simulink model "Record_accelerometer"  (R2014a)
settings: Solver=FixedStepDiscrete  StartTime=0.0  StopTime=300  FixedStep=1/400  RelTol=1e-3
undefined symbols (not defined in the file or in its folder): DiscIntNeverNeededParam
libraries: simulink x6, aerolibtransform2 x4, vrlib x3, aerolibutil x2, AR_Drone_2_Library x1, dspmtrx3 x1, Navigation_Lib x1
(part 2 of 2)

== system Record_accelerometer/Navigation Subsystem/CheckSum Pre-Processing/RateGyro Processing/CheckSum Correction ==
  CalculatedData : Inport
  CheckSumFlag : Inport  Port=2
  Holding Value : Inport  Port=3
  Compare To Zero : simulink/Logic and Bit Operations/Compare To Zero  relop=>  OutDataTypeStr=boolean
  Delay : Delay  DelayLength=3  InitialCondition=0
  Generate Sample Holding Pulse : Subsystem
  "If True, we have good data, If false, we have bad data, With bad data, use previous good data from N samples ago and hold it on that value for M samples" : Switch  Criteria=u2 > Threshold
  Invert Logic : Logic  Operator=NOT  AllPortsSameDT=off  OutDataTypeStr=boolean
  Logical Operator1 : Logic  Operator=NOT  AllPortsSameDT=off  OutDataTypeStr=boolean
  Pre-Processed Height : Outport
  wires:
  CheckSumFlag/1 -> Compare To Zero/1
  CalculatedData/1 -> "If True, we have good data, If false, we have bad data, With bad data, use previous good data from N samples ago and hold it on that value for M samples"/1
  "If True, we have good data, If false, we have bad data, With bad data, use previous good data from N samples ago and hold it on that value for M samples"/1 -> Pre-Processed Height/1, Delay/1
  Delay/1 -> "If True, we have good data, If false, we have bad data, With bad data, use previous good data from N samples ago and hold it on that value for M samples"/3
  Compare To Zero/1 -> Logical Operator1/1
  Generate Sample Holding Pulse/1(Hold_Data_Pulse) -> Invert Logic/1
  Logical Operator1/1 -> Generate Sample Holding Pulse/1(CheckSumFlag)
  Invert Logic/1 -> "If True, we have good data, If false, we have bad data, With bad data, use previous good data from N samples ago and hold it on that value for M samples"/2
  Holding Value/1 -> Generate Sample Holding Pulse/2(HoldDataTicks_Value)

== system Record_accelerometer/Navigation Subsystem/CheckSum Pre-Processing/RateGyro Processing/Process Data ==
  note: const float Sensitivity[ 3 ] = { 0.0609 , 0.0609 , 0.0609 } ;
      | const float Neutral[ 3 ] = { 0.0 , 0.0 , 0.0 } ;
      | const int16_t Offset[ 3 ] = { - 73 , 14 , - 13 } ;
      | const int16_t Noises[ 3 ] = { 35 , 35 , 15 } ;
      |
      | int16_t vRaws[ 3 ] = {
      | Navdata :: IMU :: Gyroscope :: getRawX (),
      | Navdata :: IMU :: Gyroscope :: getRawY (),
      | Navdata :: IMU :: Gyroscope :: getRawZ ()
      | } ;
      |
      | gyroscope[i] = vRaws[i] * Gyroscope :: Sensitivity[i] * M_PI / 180.0 ;
  Raw Data : Inport
  Constant : Constant  Value=[0.0, 0.0, 0.0]
  Gain : Gain  Gain=[0.0609, 0.0609, 0.0609]
  Sum : Sum  Inputs=|++
  Processed Data : Outport
  wires:
  Sum/1 -> Gain/1
  Gain/1 -> Processed Data/1
  Constant/1 -> Sum/2
  Raw Data/1 -> Sum/1

== system Record_accelerometer/Navigation Subsystem/CheckSum Pre-Processing/TempFilter/CheckSum Correction ==
  CalculatedData : Inport
  CheckSumFlag : Inport  Port=2
  Holding Value : Inport  Port=3
  Compare To Zero : simulink/Logic and Bit Operations/Compare To Zero  relop=>  OutDataTypeStr=boolean
  Delay : Delay  DelayLength=3  InitialCondition=0
  Generate Sample Holding Pulse : Subsystem
  "If True, we have good data, If false, we have bad data, With bad data, use previous good data from N samples ago and hold it on that value for M samples" : Switch  Criteria=u2 > Threshold
  Invert Logic : Logic  Operator=NOT  AllPortsSameDT=off  OutDataTypeStr=boolean
  Logical Operator1 : Logic  Operator=NOT  AllPortsSameDT=off  OutDataTypeStr=boolean
  Pre-Processed Data : Outport
  wires:
  CheckSumFlag/1 -> Compare To Zero/1
  CalculatedData/1 -> "If True, we have good data, If false, we have bad data, With bad data, use previous good data from N samples ago and hold it on that value for M samples"/1
  "If True, we have good data, If false, we have bad data, With bad data, use previous good data from N samples ago and hold it on that value for M samples"/1 -> Pre-Processed Data/1, Delay/1
  Delay/1 -> "If True, we have good data, If false, we have bad data, With bad data, use previous good data from N samples ago and hold it on that value for M samples"/3
  Compare To Zero/1 -> Logical Operator1/1
  Generate Sample Holding Pulse/1(Hold_Data_Pulse) -> Invert Logic/1
  Logical Operator1/1 -> Generate Sample Holding Pulse/1(CheckSumFlag)
  Invert Logic/1 -> "If True, we have good data, If false, we have bad data, With bad data, use previous good data from N samples ago and hold it on that value for M samples"/2
  Holding Value/1 -> Generate Sample Holding Pulse/2(HoldDataTicks_Value)

== system Record_accelerometer/Navigation Subsystem/CheckSum Pre-Processing/TempFilter/Process Raw Mag Data ==
  note: magnetometer[ 0 ] = - ( float ) navdata.mx ;
      | magnetometer[ 1 ] = ( float ) navdata.my ;
      | magnetometer[ 2 ] = - ( float ) navdata.mz ;
      | const float Sensitivity[ 3 ] = { 0.0071492608 , 0.0070882491 , 0.0074057781 } ;
      | const float Neutral[ 3 ] = { 118.0 , - 65.0 , 110.0 } ;
  Magnetometer : Inport
  Bias : Constant  Value=[ 118.0, -65.0, 110.0 ]
  Sum : Sum  Inputs=|+-
  postGain : Gain  Gain=[0.0071492608, 0.0070882491, 0.0074057781]
  preGain : Gain  Gain=[-1 1 -1]
  ProcessedData : Outport
  wires:
  postGain/1 -> ProcessedData/1
  Magnetometer/1 -> preGain/1
  Sum/1 -> postGain/1
  preGain/1 -> Sum/1
  Bias/1 -> Sum/2

== system Record_accelerometer/Navigation Subsystem/CheckSum Pre-Processing/TempFilter1/CheckSum Correction ==
  CalculatedData : Inport
  CheckSumFlag : Inport  Port=2
  Holding Value : Inport  Port=3
  Compare To Zero : simulink/Logic and Bit Operations/Compare To Zero  relop=>  OutDataTypeStr=boolean
  Delay : Delay  DelayLength=3  InitialCondition=0
  Generate Sample Holding Pulse : Subsystem
  "If True, we have good data, If false, we have bad data, With bad data, use previous good data from N samples ago and hold it on that value for M samples" : Switch  Criteria=u2 > Threshold
  Invert Logic : Logic  Operator=NOT  AllPortsSameDT=off  OutDataTypeStr=boolean
  Logical Operator1 : Logic  Operator=NOT  AllPortsSameDT=off  OutDataTypeStr=boolean
  Pre-Processed Data : Outport
  wires:
  CheckSumFlag/1 -> Compare To Zero/1
  CalculatedData/1 -> "If True, we have good data, If false, we have bad data, With bad data, use previous good data from N samples ago and hold it on that value for M samples"/1
  "If True, we have good data, If false, we have bad data, With bad data, use previous good data from N samples ago and hold it on that value for M samples"/1 -> Pre-Processed Data/1, Delay/1
  Delay/1 -> "If True, we have good data, If false, we have bad data, With bad data, use previous good data from N samples ago and hold it on that value for M samples"/3
  Compare To Zero/1 -> Logical Operator1/1
  Generate Sample Holding Pulse/1(Hold_Data_Pulse) -> Invert Logic/1
  Logical Operator1/1 -> Generate Sample Holding Pulse/1(CheckSumFlag)
  Invert Logic/1 -> "If True, we have good data, If false, we have bad data, With bad data, use previous good data from N samples ago and hold it on that value for M samples"/2
  Holding Value/1 -> Generate Sample Holding Pulse/2(HoldDataTicks_Value)

== system Record_accelerometer/Navigation Subsystem/CheckSum Pre-Processing/TempFilter1/Process Raw Mag Data ==
  note: magnetometer[ 0 ] = - ( float ) navdata.mx ;
      | magnetometer[ 1 ] = ( float ) navdata.my ;
      | magnetometer[ 2 ] = - ( float ) navdata.mz ;
      | const float Sensitivity[ 3 ] = { 0.0071492608 , 0.0070882491 , 0.0074057781 } ;
      | const float Neutral[ 3 ] = { 118.0 , - 65.0 , 110.0 } ;
  Magnetometer : Inport
  Bias : Constant  Value=[ 118.0, -65.0, 110.0 ]
  Sum : Sum  Inputs=|+-
  postGain : Gain  Gain=[0.0071492608, 0.0070882491, 0.0074057781]
  preGain : Gain  Gain=[-1 1 -1]
  ProcessedData : Outport
  wires:
  postGain/1 -> ProcessedData/1
  Magnetometer/1 -> preGain/1
  Sum/1 -> postGain/1
  preGain/1 -> Sum/1
  Bias/1 -> Sum/2

== system Record_accelerometer/Navigation Subsystem/CheckSum Pre-Processing/Ultrasound Processing/CheckSum Correction ==
  CalculatedData : Inport
  CheckSumFlag : Inport  Port=2
  Holding Value : Inport  Port=3
  Compare To Zero : simulink/Logic and Bit Operations/Compare To Zero  relop=>  OutDataTypeStr=boolean
  Delay : Delay  DelayLength=3  InitialCondition=0
  Generate Sample Holding Pulse : Subsystem
  "If True, we have good data, If false, we have bad data, With bad data, use previous good data from N samples ago and hold it on that value for M samples" : Switch  Criteria=u2 > Threshold
  Invert Logic : Logic  Operator=NOT  AllPortsSameDT=off  OutDataTypeStr=boolean
  Logical Operator1 : Logic  Operator=NOT  AllPortsSameDT=off  OutDataTypeStr=boolean
  Pre-Processed Height : Outport
  wires:
  CheckSumFlag/1 -> Compare To Zero/1
  CalculatedData/1 -> "If True, we have good data, If false, we have bad data, With bad data, use previous good data from N samples ago and hold it on that value for M samples"/1
  "If True, we have good data, If false, we have bad data, With bad data, use previous good data from N samples ago and hold it on that value for M samples"/1 -> Pre-Processed Height/1, Delay/1
  Delay/1 -> "If True, we have good data, If false, we have bad data, With bad data, use previous good data from N samples ago and hold it on that value for M samples"/3
  Compare To Zero/1 -> Logical Operator1/1
  Generate Sample Holding Pulse/1(Hold_Data_Pulse) -> Invert Logic/1
  Logical Operator1/1 -> Generate Sample Holding Pulse/1(CheckSumFlag)
  Invert Logic/1 -> "If True, we have good data, If false, we have bad data, With bad data, use previous good data from N samples ago and hold it on that value for M samples"/2
  Holding Value/1 -> Generate Sample Holding Pulse/2(HoldDataTicks_Value)

== system Record_accelerometer/Navigation Subsystem/Remove Temperature Gyro Offset/TemperatureOffset (home_330453)/Convert to Celcius ==
  In1 : Inport
  Constant1 : Constant  Value=23000  OutDataTypeStr=int16
  Data Type Conversion3 : DataTypeConversion  OutDataTypeStr=int16
  Gain1 : Gain  Gain=1/280  OutDataTypeStr=double
  Sum4 : Sum  Inputs=|++
  Out1 : Outport
  wires:
  Sum4/1 -> Gain1/1
  Gain1/1 -> Out1/1
  In1/1 -> Data Type Conversion3/1
  Data Type Conversion3/1 -> Sum4/1
  Constant1/1 -> Sum4/2

== system Record_accelerometer/Navigation Subsystem/Remove Temperature Gyro Offset/TemperatureOffset (home_330453)/Temperature Correct Pitch ==
  Temp : Inport
  Constant : Constant  Value=-293.2
  Data Type Conversion : DataTypeConversion  OutDataTypeStr=int16
  Gain1 : Gain  Commented=through  Gain=0.01074
  Gain2 : Gain  Gain=0.005239
  Sum : Sum  Inputs=|++
  Offset Correct : Outport
  wires:
  Gain2/1 -> Gain1/1
  Constant/1 -> Sum/2
  Sum/1 -> Data Type Conversion/1
  Gain1/1 -> Sum/1
  Temp/1 -> Gain2/1
  Data Type Conversion/1 -> Offset Correct/1

== system Record_accelerometer/Navigation Subsystem/Remove Temperature Gyro Offset/TemperatureOffset (home_330453)/Temperature Correct Pitch1 ==
  note: % Linear model Poly2:
      | %      f(x) = p1*x^2 + p2*x + p3
      | % Coefficients (with 95% confidence bounds):
      | %        p1 =    0.006948  (0.006782, 0.007115)
      | %        p2 =       1.056  (1.041, 1.071)
      | %        p3 =      -66.21  (-66.54, -65.88)
  Temp : Inport
  Constant1 : Constant  Value=4.961
  Gain : Gain  Gain=0.009828
  Gain3 : Gain  Gain=0.4486
  Product : Product
  Sum1 : Sum  Inputs=|+++
  Offset Correct : Outport
  wires:
  Temp/1 -> Product/1, Gain3/1, Product/2
  Product/1 -> Gain/1
  Gain/1 -> Sum1/1
  Gain3/1 -> Sum1/2
  Constant1/1 -> Sum1/3
  Sum1/1 -> Offset Correct/1

== system Record_accelerometer/Navigation Subsystem/Remove Temperature Gyro Offset/TemperatureOffset (home_330453)/Temperature Correct Roll ==
  Temp : Inport
  Data Type Conversion : DataTypeConversion  OutDataTypeStr=int16
  Offset : Constant  Value=-498.8
  Slope : Gain  Gain=0.01074
  Sum : Sum  Inputs=|++
  Offset Correction : Outport
  wires:
  Data Type Conversion/1 -> Offset Correction/1
  Offset/1 -> Sum/2
  Sum/1 -> Data Type Conversion/1  "Temperature Offset Correction"
  Slope/1 -> Sum/1
  Temp/1 -> Slope/1

== system Record_accelerometer/Navigation Subsystem/Remove Temperature Gyro Offset/TemperatureOffset (home_330453)/Temperature Correct Roll1 ==
  note: f(x) = p1*x^2 + p2*x + p3
      | Coefficients (with 95% confidence bounds):
      |        p1 =     0.01851  (0.0183, 0.01872)
      |        p2 =       1.553  (1.534, 1.572)
      |        p3 =      -13.59  (-14, -13.17)
  Temp : Inport
  Constant : Constant  Commented=on  Value=-47.33
  Constant1 : Constant  Value=-72.51+5
  Gain : Gain  Gain=-0.004462
  Gain1 : Gain  Commented=through  Gain=0.01074
  Gain2 : Gain  Commented=through  Gain=3.139
  Gain3 : Gain  Gain=1.144
  Product : Product
  Sum : Sum  Inputs=|++
  Sum1 : Sum  Inputs=|+++
  Offset Correct : Outport
  wires:
  Gain2/1 -> Gain1/1
  Constant/1 -> Sum/2
  Sum/1 -> Product/1, Gain3/1, Product/2
  Gain1/1 -> Sum/1
  Temp/1 -> Gain2/1
  Product/1 -> Gain/1
  Gain/1 -> Sum1/1
  Gain3/1 -> Sum1/2
  Constant1/1 -> Sum1/3
  Sum1/1 -> Offset Correct/1

== system Record_accelerometer/Navigation Subsystem/Remove Temperature Gyro Offset/TemperatureOffset (home_330453)/Temperature Correct Yaw ==
  Temp : Inport
  Constant : Constant  Value=-40.65
  Data Type Conversion : DataTypeConversion  OutDataTypeStr=int16
  Gain1 : Gain  Commented=through  Gain=0.01074
  Gain2 : Gain  Gain=0.0008992
  Sum : Sum  Inputs=|++
  Offset Correct : Outport
  wires:
  Gain2/1 -> Gain1/1
  Constant/1 -> Sum/2
  Sum/1 -> Data Type Conversion/1
  Gain1/1 -> Sum/1
  Temp/1 -> Gain2/1
  Data Type Conversion/1 -> Offset Correct/1

== system Record_accelerometer/Navigation Subsystem/Remove Temperature Gyro Offset/TemperatureOffset (home_330453)/Temperature Correct Yaw1 ==
  note: f(x) = p1*x^2 + p2*x + p3
      | Coefficients (with 95% confidence bounds):
      |        p1 =     0.01851  (0.0183, 0.01872)
      |        p2 =       1.553  (1.534, 1.572)
      |        p3 =      -13.59  (-14, -13.17)
  note: f(x) = p1*x^2 + p2*x + p3
      | Coefficients (with 95% confidence bounds):
      |        p1 =    -0.00233  (-0.002509, -0.00215)
      |        p2 =        0.46  (0.444, 0.476)
      |        p3 =      -7.059  (-7.413, -6.705)
  Temp : Inport
  Constant : Constant  Commented=on  Value=-47.33
  Constant1 : Constant  Value=-7.059
  Gain : Gain  Gain=-0.00233
  Gain1 : Gain  Commented=through  Gain=0.01074
  Gain2 : Gain  Commented=through  Gain=3.139
  Gain3 : Gain  Gain=0.46
  Product : Product
  Sum : Sum  Inputs=|++
  Sum1 : Sum  Inputs=|+++
  Offset Correct : Outport
  wires:
  Gain2/1 -> Gain1/1
  Constant/1 -> Sum/2
  Sum/1 -> Product/1, Gain3/1, Product/2
  Gain1/1 -> Sum/1
  Temp/1 -> Gain2/1
  Product/1 -> Gain/1
  Gain/1 -> Sum1/1
  Gain3/1 -> Sum1/2
  Constant1/1 -> Sum1/3
  Sum1/1 -> Offset Correct/1

== system Record_accelerometer/Navigation Subsystem/Remove Temperature Gyro Offset/TemperatureOffset (work_255725)/Convert to Celcius ==
  In1 : Inport
  Constant1 : Constant  Value=23000  OutDataTypeStr=int16
  Data Type Conversion3 : DataTypeConversion  OutDataTypeStr=int16
  Gain1 : Gain  Gain=1/280  OutDataTypeStr=double
  Sum4 : Sum  Inputs=|++
  Out1 : Outport
  wires:
  Sum4/1 -> Gain1/1
  Gain1/1 -> Out1/1
  In1/1 -> Data Type Conversion3/1
  Data Type Conversion3/1 -> Sum4/1
  Constant1/1 -> Sum4/2

== system Record_accelerometer/Navigation Subsystem/Remove Temperature Gyro Offset/TemperatureOffset (work_255725)/Temperature Correct Pitch ==
  Temp : Inport
  Constant : Constant  Value=-293.2
  Data Type Conversion : DataTypeConversion  OutDataTypeStr=int16
  Gain1 : Gain  Commented=through  Gain=0.01074
  Gain2 : Gain  Gain=0.005239
  Sum : Sum  Inputs=|++
  Offset Correct : Outport
  wires:
  Gain2/1 -> Gain1/1
  Constant/1 -> Sum/2
  Sum/1 -> Data Type Conversion/1
  Gain1/1 -> Sum/1
  Temp/1 -> Gain2/1
  Data Type Conversion/1 -> Offset Correct/1

== system Record_accelerometer/Navigation Subsystem/Remove Temperature Gyro Offset/TemperatureOffset (work_255725)/Temperature Correct Pitch1 ==
  note: % Linear model Poly2:
      | %      f(x) = p1*x^2 + p2*x + p3
      | % Coefficients (with 95% confidence bounds):
      | %        p1 =    0.006948  (0.006782, 0.007115)
      | %        p2 =       1.056  (1.041, 1.071)
      | %        p3 =      -66.21  (-66.54, -65.88)
  Temp : Inport
  Constant1 : Constant  Value=-66.21
  Gain : Gain  Gain=0.006948
  Gain3 : Gain  Gain=1.056
  Product : Product
  Sum1 : Sum  Inputs=|+++
  Offset Correct : Outport
  wires:
  Temp/1 -> Product/1, Gain3/1, Product/2
  Product/1 -> Gain/1
  Gain/1 -> Sum1/1
  Gain3/1 -> Sum1/2
  Constant1/1 -> Sum1/3
  Sum1/1 -> Offset Correct/1

== system Record_accelerometer/Navigation Subsystem/Remove Temperature Gyro Offset/TemperatureOffset (work_255725)/Temperature Correct Roll ==
  Temp : Inport
  Data Type Conversion : DataTypeConversion  OutDataTypeStr=int16
  Offset : Constant  Value=-498.8
  Slope : Gain  Gain=0.01074
  Sum : Sum  Inputs=|++
  Offset Correction : Outport
  wires:
  Data Type Conversion/1 -> Offset Correction/1
  Offset/1 -> Sum/2
  Sum/1 -> Data Type Conversion/1  "Temperature Offset Correction"
  Slope/1 -> Sum/1
  Temp/1 -> Slope/1

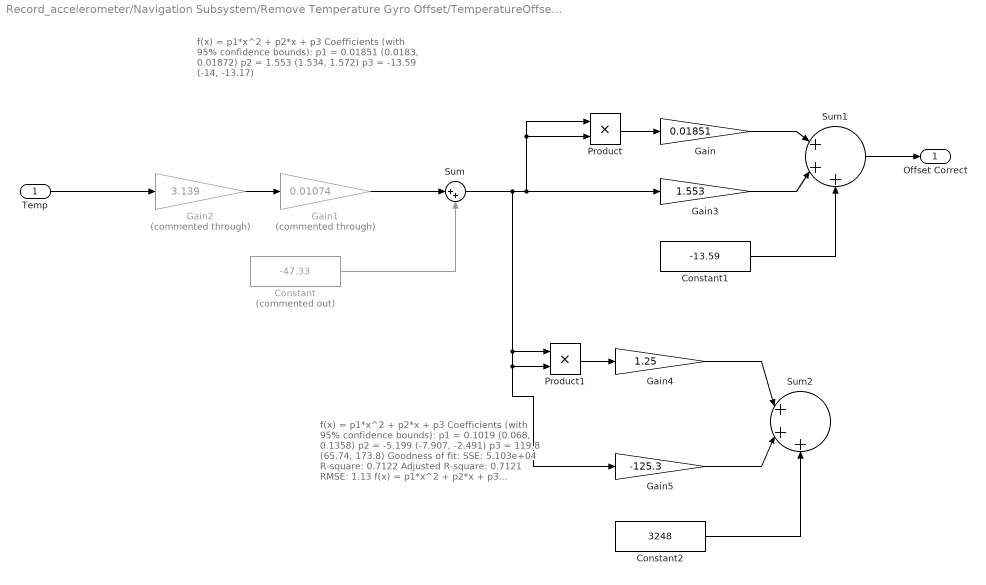
== system Record_accelerometer/Navigation Subsystem/Remove Temperature Gyro Offset/TemperatureOffset (work_255725)/Temperature Correct Roll1 ==
  note: f(x) = p1*x^2 + p2*x + p3
      | Coefficients (with 95% confidence bounds):
      |        p1 =      0.1019  (0.068, 0.1358)
      |        p2 =      -5.199  (-7.907, -2.491)
      |        p3 =       119.8  (65.74, 173.8)
      |
      | Goodness of fit:
      |   SSE: 5.103e+04
      |   R-square: 0.7122
      |   Adjusted R-square: 0.7121
      |   RMSE: 1.13
      |
      |
      |      f(x) = p1*x^2 + p2*x + p3
      | Coefficients (with 95% confidence bounds):
      |        p1 =        1.25  (1.214, 1.287)
      |        p2 =      -125.3  (-129.1, -121.5)
      |        p3 =        3248  (3149, 3347)
  note: f(x) = p1*x^2 + p2*x + p3
      | Coefficients (with 95% confidence bounds):
      |        p1 =     0.01851  (0.0183, 0.01872)
      |        p2 =       1.553  (1.534, 1.572)
      |        p3 =      -13.59  (-14, -13.17)
  Temp : Inport
  Constant : Constant  Commented=on  Value=-47.33
  Constant1 : Constant  Value=-13.59
  Constant2 : Constant  Value=3248
  Gain : Gain  Gain=0.01851
  Gain1 : Gain  Commented=through  Gain=0.01074
  Gain2 : Gain  Commented=through  Gain=3.139
  Gain3 : Gain  Gain=1.553
  Gain4 : Gain  Gain=1.25
  Gain5 : Gain  Gain=-125.3
  Product : Product
  Product1 : Product
  Sum : Sum  Inputs=|++
  Sum1 : Sum  Inputs=|+++
  Sum2 : Sum  Inputs=|+++
  Offset Correct : Outport
  wires:
  Gain2/1 -> Gain1/1
  Constant/1 -> Sum/2
  Sum/1 -> Product/2, Product/1, Gain3/1, Product1/1, Gain5/1, Product1/2
  Gain1/1 -> Sum/1
  Temp/1 -> Gain2/1
  Product/1 -> Gain/1
  Gain/1 -> Sum1/1
  Gain3/1 -> Sum1/2
  Constant1/1 -> Sum1/3
  Gain4/1 -> Sum2/1
  Gain5/1 -> Sum2/2
  Constant2/1 -> Sum2/3
  Product1/1 -> Gain4/1
  Sum1/1 -> Offset Correct/1

== system Record_accelerometer/Navigation Subsystem/Remove Temperature Gyro Offset/TemperatureOffset (work_255725)/Temperature Correct Yaw ==
  Temp : Inport
  Constant : Constant  Value=-40.65
  Data Type Conversion : DataTypeConversion  OutDataTypeStr=int16
  Gain1 : Gain  Commented=through  Gain=0.01074
  Gain2 : Gain  Gain=0.0008992
  Sum : Sum  Inputs=|++
  Offset Correct : Outport
  wires:
  Gain2/1 -> Gain1/1
  Constant/1 -> Sum/2
  Sum/1 -> Data Type Conversion/1
  Gain1/1 -> Sum/1
  Temp/1 -> Gain2/1
  Data Type Conversion/1 -> Offset Correct/1

== system Record_accelerometer/Navigation Subsystem/Remove Temperature Gyro Offset/TemperatureOffset (work_255725)/Temperature Correct Yaw1 ==
  note: f(x) = p1*x^2 + p2*x + p3
      | Coefficients (with 95% confidence bounds):
      |        p1 =     0.01851  (0.0183, 0.01872)
      |        p2 =       1.553  (1.534, 1.572)
      |        p3 =      -13.59  (-14, -13.17)
  note: f(x) = p1*x^2 + p2*x + p3
      | Coefficients (with 95% confidence bounds):
      |        p1 =    -0.00233  (-0.002509, -0.00215)
      |        p2 =        0.46  (0.444, 0.476)
      |        p3 =      -7.059  (-7.413, -6.705)
  Temp : Inport
  Constant : Constant  Commented=on  Value=-47.33
  Constant1 : Constant  Value=-7.962
  Gain : Gain  Gain=0.009834
  Gain1 : Gain  Commented=through  Gain=0.01074
  Gain2 : Gain  Commented=through  Gain=3.139
  Gain3 : Gain  Gain=-0.4009
  Product : Product
  Sum : Sum  Inputs=|++
  Sum1 : Sum  Inputs=|+++
  Offset Correct : Outport
  wires:
  Gain2/1 -> Gain1/1
  Constant/1 -> Sum/2
  Sum/1 -> Product/1, Gain3/1, Product/2
  Gain1/1 -> Sum/1
  Temp/1 -> Gain2/1
  Product/1 -> Gain/1
  Gain/1 -> Sum1/1
  Gain3/1 -> Sum1/2
  Constant1/1 -> Sum1/3
  Sum1/1 -> Offset Correct/1

== system Record_accelerometer/Navigation Subsystem/Remove Temperature Gyro Offset/TemperatureOffset (work_255725)/Temperature Correct Yaw2 ==
  note: f(x) = p1*x^2 + p2*x + p3
      | Coefficients (with 95% confidence bounds):
      |        p1 =     0.01851  (0.0183, 0.01872)
      |        p2 =       1.553  (1.534, 1.572)
      |        p3 =      -13.59  (-14, -13.17)
  note: f(x) = p1*x^2 + p2*x + p3
      | Coefficients (with 95% confidence bounds):
      |        p1 =    -0.00233  (-0.002509, -0.00215)
      |        p2 =        0.46  (0.444, 0.476)
      |        p3 =      -7.059  (-7.413, -6.705)
  Temp : Inport
  Constant : Constant  Commented=on  Value=-47.33
  Constant1 : Constant  Value=-7.059
  Gain : Gain  Gain=-0.00233
  Gain1 : Gain  Commented=through  Gain=0.01074
  Gain2 : Gain  Commented=through  Gain=3.139
  Gain3 : Gain  Gain=0.46
  Product : Product
  Sum : Sum  Inputs=|++
  Sum1 : Sum  Inputs=|+++
  Offset Correct : Outport
  wires:
  Gain2/1 -> Gain1/1
  Constant/1 -> Sum/2
  Sum/1 -> Product/1, Gain3/1, Product/2
  Gain1/1 -> Sum/1
  Temp/1 -> Gain2/1
  Product/1 -> Gain/1
  Gain/1 -> Sum1/1
  Gain3/1 -> Sum1/2
  Constant1/1 -> Sum1/3
  Sum1/1 -> Offset Correct/1

== system Record_accelerometer/Navigation Subsystem/SL3D Visualization/Interchange Axes Mag for SL3D /Home Drone ==
  note: This comes close, however, it doesnt seem that the axis changes properly
      | ie: i rotate drone, the green dot follows it. This  tells me the Z-axis is not
      |  properly placed
  note: y
  note: x
  note: z
  In1 : Inport
  Demux1 : Demux  Outputs=3
  Gain : Gain  Gain=-1
  Gain1 : Gain
  Gain2 : Gain
  Mux2 : Mux  Inputs=3
  Out1 : Outport
  wires:
  Mux2/1 -> Out1/1
  In1/1 -> Demux1/1
  Demux1/3 -> Gain2/1
  Gain2/1 -> Mux2/2
  Demux1/1 -> Gain/1
  Gain/1 -> Mux2/3
  Demux1/2 -> Gain1/1
  Gain1/1 -> Mux2/1

== system Record_accelerometer/Navigation Subsystem/SL3D Visualization/Interchange Axes Mag for SL3D /Subsystem ==
  note: This comes close, however, it doesnt seem that the axis changes properly
      | ie: i rotate drone, the green dot follows it. This  tells me the Z-axis is not
      |  properly placed
  note: y
  note: x
  note: z
  In1 : Inport
  Demux1 : Demux  Outputs=3
  Gain : Gain
  Gain1 : Gain  Gain=-1
  Gain2 : Gain  Gain=-1
  Mux2 : Mux  Inputs=3
  Out1 : Outport
  wires:
  Demux1/1 -> Gain2/1
  Gain2/1 -> Mux2/2
  Gain/1 -> Mux2/3
  Gain1/1 -> Mux2/1
  Mux2/1 -> Out1/1
  Demux1/2 -> Gain1/1
  Demux1/3 -> Gain/1
  In1/1 -> Demux1/1

== system Record_accelerometer/Navigation Subsystem/SL3D Visualization/Interchange Axes Mag for SL3D /Work Drone ==
  note: This comes close, however, it doesnt seem that the axis changes properly
      | ie: i rotate drone, the green dot follows it. This  tells me the Z-axis is not
      |  properly placed
  note: y
  note: x
  note: z
  In1 : Inport
  Demux1 : Demux  Outputs=3
  Gain : Gain  Gain=-1
  Gain1 : Gain
  Gain2 : Gain
  Mux2 : Mux  Inputs=3
  Out1 : Outport
  wires:
  Mux2/1 -> Out1/1
  In1/1 -> Demux1/1
  Demux1/3 -> Gain2/1
  Gain2/1 -> Mux2/2
  Demux1/1 -> Gain/1
  Gain/1 -> Mux2/3
  Demux1/2 -> Gain1/1
  Gain1/1 -> Mux2/1

== system Record_accelerometer/Navigation Subsystem/SL3D Visualization/Interchange Axes Mag for SL3D /Work Drone - supposed work drone .. not really ==
  note: This comes close, however, it doesnt seem that the axis changes properly
      | ie: i rotate drone, the green dot follows it. This  tells me the Z-axis is not
      |  properly placed
  note: y
  note: x
  note: z
  In1 : Inport
  Demux1 : Demux  Outputs=3
  Gain : Gain  Gain=-1
  Gain1 : Gain
  Gain2 : Gain  Gain=-1
  Mux2 : Mux  Inputs=3
  Out1 : Outport
  wires:
  Mux2/1 -> Out1/1
  In1/1 -> Demux1/1
  Demux1/3 -> Gain2/1
  Gain2/1 -> Mux2/2
  Demux1/1 -> Gain/1
  Gain/1 -> Mux2/3
  Demux1/2 -> Gain1/1
  Gain1/1 -> Mux2/1

== system Record_accelerometer/Navigation Subsystem/CheckSum Pre-Processing/Accelerometer Processing/CheckSum Correction/Generate Sample Holding Pulse ==
  CheckSumFlag : Inport
  HoldDataTicks_Value : Inport  Port=2
  Chart : Stateflow chart  TreatAsAtomicUnit=on
  Constant2 : Constant
  Logical Operator1 : Logic  AllPortsSameDT=off  OutDataTypeStr=boolean
  Transition Logic Detection : Subsystem
  Hold_Data_Pulse : Outport
  wires:
  Constant2/1 -> Logical Operator1/1
  Logical Operator1/1 -> Hold_Data_Pulse/1
  Chart/1(output) -> Logical Operator1/2
  Transition Logic Detection/1(Transition Detect) -> Chart/1(if_transition)
  CheckSumFlag/1 -> Transition Logic Detection/1(Input)
  HoldDataTicks_Value/1 -> Chart/2(HoldDataTicks)

== system Record_accelerometer/Navigation Subsystem/CheckSum Pre-Processing/Magnetometer/CheckSum Correction/Generate Sample Holding Pulse ==
  CheckSumFlag : Inport
  HoldDataTicks_Value : Inport  Port=2
  Chart : Stateflow chart  TreatAsAtomicUnit=on
  Constant2 : Constant
  Logical Operator1 : Logic  AllPortsSameDT=off  OutDataTypeStr=boolean
  Transition Logic Detection : Subsystem
  Hold_Data_Pulse : Outport
  wires:
  Constant2/1 -> Logical Operator1/1
  Logical Operator1/1 -> Hold_Data_Pulse/1
  Chart/1(output) -> Logical Operator1/2
  Transition Logic Detection/1(Transition Detect) -> Chart/1(if_transition)
  CheckSumFlag/1 -> Transition Logic Detection/1(Input)
  HoldDataTicks_Value/1 -> Chart/2(HoldDataTicks)

== system Record_accelerometer/Navigation Subsystem/CheckSum Pre-Processing/RateGyro Processing/CheckSum Correction/Generate Sample Holding Pulse ==
  CheckSumFlag : Inport
  HoldDataTicks_Value : Inport  Port=2
  Chart : Stateflow chart  TreatAsAtomicUnit=on
  Constant2 : Constant
  Logical Operator1 : Logic  AllPortsSameDT=off  OutDataTypeStr=boolean
  Transition Logic Detection : Subsystem
  Hold_Data_Pulse : Outport
  wires:
  Constant2/1 -> Logical Operator1/1
  Logical Operator1/1 -> Hold_Data_Pulse/1
  Chart/1(output) -> Logical Operator1/2
  Transition Logic Detection/1(Transition Detect) -> Chart/1(if_transition)
  CheckSumFlag/1 -> Transition Logic Detection/1(Input)
  HoldDataTicks_Value/1 -> Chart/2(HoldDataTicks)

== system Record_accelerometer/Navigation Subsystem/CheckSum Pre-Processing/TempFilter/CheckSum Correction/Generate Sample Holding Pulse ==
  CheckSumFlag : Inport
  HoldDataTicks_Value : Inport  Port=2
  Chart : Stateflow chart  TreatAsAtomicUnit=on
  Constant2 : Constant
  Logical Operator1 : Logic  AllPortsSameDT=off  OutDataTypeStr=boolean
  Transition Logic Detection : Subsystem
  Hold_Data_Pulse : Outport
  wires:
  Constant2/1 -> Logical Operator1/1
  Logical Operator1/1 -> Hold_Data_Pulse/1
  Chart/1(output) -> Logical Operator1/2
  Transition Logic Detection/1(Transition Detect) -> Chart/1(if_transition)
  CheckSumFlag/1 -> Transition Logic Detection/1(Input)
  HoldDataTicks_Value/1 -> Chart/2(HoldDataTicks)

== system Record_accelerometer/Navigation Subsystem/CheckSum Pre-Processing/TempFilter1/CheckSum Correction/Generate Sample Holding Pulse ==
  CheckSumFlag : Inport
  HoldDataTicks_Value : Inport  Port=2
  Chart : Stateflow chart  TreatAsAtomicUnit=on
  Constant2 : Constant
  Logical Operator1 : Logic  AllPortsSameDT=off  OutDataTypeStr=boolean
  Transition Logic Detection : Subsystem
  Hold_Data_Pulse : Outport
  wires:
  Constant2/1 -> Logical Operator1/1
  Logical Operator1/1 -> Hold_Data_Pulse/1
  Chart/1(output) -> Logical Operator1/2
  Transition Logic Detection/1(Transition Detect) -> Chart/1(if_transition)
  CheckSumFlag/1 -> Transition Logic Detection/1(Input)
  HoldDataTicks_Value/1 -> Chart/2(HoldDataTicks)

== system Record_accelerometer/Navigation Subsystem/CheckSum Pre-Processing/Ultrasound Processing/CheckSum Correction/Generate Sample Holding Pulse ==
  CheckSumFlag : Inport
  HoldDataTicks_Value : Inport  Port=2
  Chart : Stateflow chart  TreatAsAtomicUnit=on
  Constant2 : Constant
  Logical Operator1 : Logic  AllPortsSameDT=off  OutDataTypeStr=boolean
  Transition Logic Detection : Subsystem
  Hold_Data_Pulse : Outport
  wires:
  Constant2/1 -> Logical Operator1/1
  Logical Operator1/1 -> Hold_Data_Pulse/1
  Chart/1(output) -> Logical Operator1/2
  Transition Logic Detection/1(Transition Detect) -> Chart/1(if_transition)
  CheckSumFlag/1 -> Transition Logic Detection/1(Input)
  HoldDataTicks_Value/1 -> Chart/2(HoldDataTicks)

== system Record_accelerometer/Navigation Subsystem/CheckSum Pre-Processing/Accelerometer Processing/CheckSum Correction/Generate Sample Holding Pulse/Transition Logic Detection ==
  Input : Inport
  Constant : Constant  Value=0
  Constant1 : Constant
  Logical Operator : Logic  AllPortsSameDT=off  OutDataTypeStr=boolean
  Relational Operator : RelationalOperator  Operator===  OutDataTypeStr=boolean
  Relational Operator1 : RelationalOperator  Operator===  OutDataTypeStr=boolean
  Unit Delay : UnitDelay  SampleTime=-1
  Transition Detect : Outport
  wires:
  Relational Operator1/1 -> Logical Operator/1
  Unit Delay/1 -> Relational Operator/1
  Input/1 -> Relational Operator1/2, Unit Delay/1
  Relational Operator/1 -> Logical Operator/2
  Constant/1 -> Relational Operator/2
  Constant1/1 -> Relational Operator1/1
  Logical Operator/1 -> Transition Detect/1  "Transition_Detect"

== system Record_accelerometer/Navigation Subsystem/CheckSum Pre-Processing/Magnetometer/CheckSum Correction/Generate Sample Holding Pulse/Transition Logic Detection ==
  Input : Inport
  Constant : Constant  Value=0
  Constant1 : Constant
  Logical Operator : Logic  AllPortsSameDT=off  OutDataTypeStr=boolean
  Relational Operator : RelationalOperator  Operator===  OutDataTypeStr=boolean
  Relational Operator1 : RelationalOperator  Operator===  OutDataTypeStr=boolean
  Unit Delay : UnitDelay  SampleTime=-1
  Transition Detect : Outport
  wires:
  Relational Operator1/1 -> Logical Operator/1
  Unit Delay/1 -> Relational Operator/1
  Input/1 -> Relational Operator1/2, Unit Delay/1
  Relational Operator/1 -> Logical Operator/2
  Constant/1 -> Relational Operator/2
  Constant1/1 -> Relational Operator1/1
  Logical Operator/1 -> Transition Detect/1  "Transition_Detect"

== system Record_accelerometer/Navigation Subsystem/CheckSum Pre-Processing/RateGyro Processing/CheckSum Correction/Generate Sample Holding Pulse/Transition Logic Detection ==
  Input : Inport
  Constant : Constant  Value=0
  Constant1 : Constant
  Logical Operator : Logic  AllPortsSameDT=off  OutDataTypeStr=boolean
  Relational Operator : RelationalOperator  Operator===  OutDataTypeStr=boolean
  Relational Operator1 : RelationalOperator  Operator===  OutDataTypeStr=boolean
  Unit Delay : UnitDelay  SampleTime=-1
  Transition Detect : Outport
  wires:
  Relational Operator1/1 -> Logical Operator/1
  Unit Delay/1 -> Relational Operator/1
  Input/1 -> Relational Operator1/2, Unit Delay/1
  Relational Operator/1 -> Logical Operator/2
  Constant/1 -> Relational Operator/2
  Constant1/1 -> Relational Operator1/1
  Logical Operator/1 -> Transition Detect/1  "Transition_Detect"

== system Record_accelerometer/Navigation Subsystem/CheckSum Pre-Processing/TempFilter/CheckSum Correction/Generate Sample Holding Pulse/Transition Logic Detection ==
  Input : Inport
  Constant : Constant  Value=0
  Constant1 : Constant
  Logical Operator : Logic  AllPortsSameDT=off  OutDataTypeStr=boolean
  Relational Operator : RelationalOperator  Operator===  OutDataTypeStr=boolean
  Relational Operator1 : RelationalOperator  Operator===  OutDataTypeStr=boolean
  Unit Delay : UnitDelay  SampleTime=-1
  Transition Detect : Outport
  wires:
  Relational Operator1/1 -> Logical Operator/1
  Unit Delay/1 -> Relational Operator/1
  Input/1 -> Relational Operator1/2, Unit Delay/1
  Relational Operator/1 -> Logical Operator/2
  Constant/1 -> Relational Operator/2
  Constant1/1 -> Relational Operator1/1
  Logical Operator/1 -> Transition Detect/1  "Transition_Detect"

== system Record_accelerometer/Navigation Subsystem/CheckSum Pre-Processing/TempFilter1/CheckSum Correction/Generate Sample Holding Pulse/Transition Logic Detection ==
  Input : Inport
  Constant : Constant  Value=0
  Constant1 : Constant
  Logical Operator : Logic  AllPortsSameDT=off  OutDataTypeStr=boolean
  Relational Operator : RelationalOperator  Operator===  OutDataTypeStr=boolean
  Relational Operator1 : RelationalOperator  Operator===  OutDataTypeStr=boolean
  Unit Delay : UnitDelay  SampleTime=-1
  Transition Detect : Outport
  wires:
  Relational Operator1/1 -> Logical Operator/1
  Unit Delay/1 -> Relational Operator/1
  Input/1 -> Relational Operator1/2, Unit Delay/1
  Relational Operator/1 -> Logical Operator/2
  Constant/1 -> Relational Operator/2
  Constant1/1 -> Relational Operator1/1
  Logical Operator/1 -> Transition Detect/1  "Transition_Detect"

== system Record_accelerometer/Navigation Subsystem/CheckSum Pre-Processing/Ultrasound Processing/CheckSum Correction/Generate Sample Holding Pulse/Transition Logic Detection ==
  Input : Inport
  Constant : Constant  Value=0
  Constant1 : Constant
  Logical Operator : Logic  AllPortsSameDT=off  OutDataTypeStr=boolean
  Relational Operator : RelationalOperator  Operator===  OutDataTypeStr=boolean
  Relational Operator1 : RelationalOperator  Operator===  OutDataTypeStr=boolean
  Unit Delay : UnitDelay  SampleTime=-1
  Transition Detect : Outport
  wires:
  Relational Operator1/1 -> Logical Operator/1
  Unit Delay/1 -> Relational Operator/1
  Input/1 -> Relational Operator1/2, Unit Delay/1
  Relational Operator/1 -> Logical Operator/2
  Constant/1 -> Relational Operator/2
  Constant1/1 -> Relational Operator1/1
  Logical Operator/1 -> Transition Detect/1  "Transition_Detect"

== matlab function Record_accelerometer/Navigation Subsystem/CheckSum Pre-Processing/Ultrasound Processing/Height Calculation ==
  data: u input double; y output double; prev_good_height output double; z_1 input double
function [y,prev_good_height] = fcn(u,z_1)
%#codegen



if u<10000
    
    height = ((u - 880) /26.553);
    prev_good_height = height;
else
    
%     height = u;
%     prev_good_height = height;
    height =  z_1;
    prev_good_height = z_1; 
end

y = height;

== stateflow chart Record_accelerometer/Navigation Subsystem/CheckSum Pre-Processing/Accelerometer Processing/CheckSum Correction/Generate Sample Holding Pulse/Chart ==
  state Begin_State0
    entry: output =0;
  state Begin_State
    entry: output =1;
  state End_State
    entry: output=0;
  (default) -> Begin_State0
  Begin_State0 -> Begin_State : [if_transition==1]
  Begin_State -> End_State [order 1] : after(HoldDataTicks,tick)
  End_State -> Begin_State : [if_transition==1]
  Begin_State -> Begin_State [order 2] : [if_transition==1]
  data: output output; if_transition input; HoldDataTicks input

== stateflow chart Record_accelerometer/Navigation Subsystem/CheckSum Pre-Processing/RateGyro Processing/CheckSum Correction/Generate Sample Holding Pulse/Chart ==
  state Begin_State0
    entry: output =0;
  state Begin_State
    entry: output =1;
  state End_State
    entry: output=0;
  (default) -> Begin_State0
  Begin_State0 -> Begin_State : [if_transition==1]
  Begin_State -> End_State [order 1] : after(HoldDataTicks,tick)
  End_State -> Begin_State : [if_transition==1]
  Begin_State -> Begin_State [order 2] : [if_transition==1]
  data: output output; if_transition input; HoldDataTicks input

== stateflow chart Record_accelerometer/Navigation Subsystem/CheckSum Pre-Processing/Ultrasound Processing/CheckSum Correction/Generate Sample Holding Pulse/Chart ==
  state Begin_State0
    entry: output =0;
  state Begin_State
    entry: output =1;
  state End_State
    entry: output=0;
  (default) -> Begin_State0
  Begin_State0 -> Begin_State : [if_transition==1]
  Begin_State -> End_State [order 1] : after(HoldDataTicks,tick)
  End_State -> Begin_State : [if_transition==1]
  Begin_State -> Begin_State [order 2] : [if_transition==1]
  data: output output; if_transition input; HoldDataTicks input

== stateflow chart Record_accelerometer/Navigation Subsystem/CheckSum Pre-Processing/Magnetometer/CheckSum Correction/Generate Sample Holding Pulse/Chart ==
  state Begin_State0
    entry: output =0;
  state Begin_State
    entry: output =1;
  state End_State
    entry: output=0;
  (default) -> Begin_State0
  Begin_State0 -> Begin_State : [if_transition==1]
  Begin_State -> End_State [order 1] : after(HoldDataTicks,tick)
  End_State -> Begin_State : [if_transition==1]
  Begin_State -> Begin_State [order 2] : [if_transition==1]
  data: output output; if_transition input; HoldDataTicks input

== stateflow chart Record_accelerometer/Navigation Subsystem/CheckSum Pre-Processing/TempFilter1/CheckSum Correction/Generate Sample Holding Pulse/Chart ==
  state Begin_State0
    entry: output =0;
  state Begin_State
    entry: output =1;
  state End_State
    entry: output=0;
  (default) -> Begin_State0
  Begin_State0 -> Begin_State : [if_transition==1]
  Begin_State -> End_State [order 1] : after(HoldDataTicks,tick)
  End_State -> Begin_State : [if_transition==1]
  Begin_State -> Begin_State [order 2] : [if_transition==1]
  data: output output; if_transition input; HoldDataTicks input

== stateflow chart Record_accelerometer/Navigation Subsystem/CheckSum Pre-Processing/TempFilter/CheckSum Correction/Generate Sample Holding Pulse/Chart ==
  state Begin_State0
    entry: output =0;
  state Begin_State
    entry: output =1;
  state End_State
    entry: output=0;
  (default) -> Begin_State0
  Begin_State0 -> Begin_State : [if_transition==1]
  Begin_State -> End_State [order 1] : after(HoldDataTicks,tick)
  End_State -> Begin_State : [if_transition==1]
  Begin_State -> Begin_State [order 2] : [if_transition==1]
  data: output output; if_transition input; HoldDataTicks input

== matlab function Record_accelerometer/Navigation Subsystem/SL3D Visualization/Matrix Re-Order ==
  data: M_in input; M_out output
function M_out = MatrixFormat(M_in)
%#codegen

% SL3D coordinate system is different. This EML block is responsible for
% re-ordering the matrix in a format that SL3D can understand

M_out = M_in ; %set size

%re-order diagonal
M_out(1,1) = M_in(2,2);
M_out(2,2) = M_in(3,3);
M_out(3,3) = M_in(1,1);

%re-order bottom half
M_out(2,1) = M_in(3,2) ;
M_out(3,1) = M_in(1,2) ;
M_out(3,2) = M_in(1,3);

%re-order upper half
M_out(1,2) = M_in(2,3);
M_out(1,3) = M_in(2,1) ;
M_out(2,3) = M_in(3,1);

== matlab function Record_accelerometer/Navigation Subsystem/KF_YAW/Kalman Tracker ==
  data: prev_state input; covariance_correction_prev input; state_correction output; covariance_correction output; ctrl_input_gyro input; measurement_angle input
function [state_correction, covariance_correction] = fcn(prev_state, covariance_correction_prev, ctrl_input_gyro, measurement_angle)


%-------------------------------
%-------------------------------
%---- Predict Stage ------------
%-------------------------------
%-------------------------------
% pix_value = 5;
Ts = 1/400;
%Process Noise
p_var =0.01;
Q = [p_var^2     0         
      0         p_var^2];

%A matrix
A =  [1   -Ts 
      0   1];

%odutput these values with a unit delay (for algebraic loop), apply initial conditions
state_prediction = A*prev_state + [Ts 0; 0 0]*[ctrl_input_gyro; 0 ];
covariance_prediction = A*covariance_correction_prev*A' + Q;

%-------------------------------
%-------------------------------
%---- Estimate Stage -----------
%-------------------------------
%-------------------------------

    %H matrix
    H = [1 0];

    %Measurement noise from accelerometer angle measurement
    m_var = 1;
%     m_var_r = 1;

    R = [m_var^2 ];

    %Measurement Z
    Z = [measurement_angle];

    %Compute Kalman Gain
    Kalman_Gain = covariance_prediction*H'*inv(H*covariance_prediction*H'+R); %2x2 matrix

    %compute state space correction based on measurement
    state_correction = state_prediction + Kalman_Gain*(Z - H*state_prediction); %4x1 vector of states

    %compute covariance correction
    covariance_correction = (eye(2) - Kalman_Gain*H)*covariance_prediction; %2x2 covariance matrix

%     corrected_angle_measure = state_correction(1) - Ts*state_correction(2);
end

== matlab function Record_accelerometer/Navigation Subsystem/Calculate Roll - Pitch/MATLAB Function ==
  data: Ax_Ay_Az input; Roll output; Pitch output
function [Roll,Pitch] = CalculateAngle(Ax_Ay_Az)
%#codegen
Ax = -Ax_Ay_Az(1);
Ay = -Ax_Ay_Az(2);
Az = Ax_Ay_Az(3);

Pitch = atan( Ax / sqrt( Ay^2 + Az^2));
Roll = atan( Ay / sqrt( Ax^2 + Az^2));

== matlab function Record_accelerometer/Navigation Subsystem/SL3D Visualization/Subsystem/Compensate for Magnetic Declination (~60 degrees in Boston)_ ==
  data: vector_in input; y output
function y = fcn(vector_in)
%#codegen

% %  WHY WAS THIS COMMENTED OUT???
% %  Reason: While the intention to rotate 60 degrees up north was in good
% %  intention, the math was not correct: you are rotating in the global
% %  reference frame, an axis which stays fixed. we want to rotate upwards
% %  along an axis which is perpindicular to the XY coordinates
% %

%transform the pitch up, recall that in SL3D the x-axis = z-axis
%                                                y-axis = x-axis

rotation = 1*pi/3;
C_term = cos(rotation);
S_term = sin(rotation);
MatrixY = [C_term 0 -S_term; 0 1 0; S_term 0 C_term ];
MatrixX = [1 0 0; 0 C_term -S_term; 0 S_term C_term ];


y = MatrixY*vector_in;

== matlab function Record_accelerometer/Navigation Subsystem/SL3D Visualization/Subsystem/Compensate for Magnetic Declination (~60 degrees in Boston)_1 ==
  data: vector_in input; y output
function y = fcn(vector_in)
%#codegen


Declination_Angle = 1*pi/3;

rot_axis = [vector_in(2) -vector_in(1)]; %find a vector perpindicular to the XY vector, such that we can pitch around it
rot_axis = rot_axis/norm(rot_axis);
%rotate by this amount
% for i=1:1:45;
% rot_angle = i*(pi/180) ;

%Define new rotation matrix
C_term = cos(Declination_Angle);
S_term = sin(Declination_Angle);
t = 1-C_term;
ux = rot_axis(1);
uy = rot_axis(2);
uz = 0; 

new_rot = [(t*ux^2 + C_term) (t*ux*uy-S_term*uz) (t*ux*uz+S_term*uy)
           (t*ux*uy+S_term*uz) (t*uy^2+C_term)     (t*uy*uz - S_term*ux)
           (t*ux*uz - S_term*uy) (t*uy*uz+S_term*ux) (t*uz^2 + C_term)];


y = new_rot*vector_in;

== matlab function Record_accelerometer/Navigation Subsystem/KF_ROLL/Kalman Tracker ==
  data: prev_state input; covariance_correction_prev input; state_correction output; covariance_correction output; ctrl_input_gyro input; measurement_angle input
function [state_correction, covariance_correction] = fcn(prev_state, covariance_correction_prev, ctrl_input_gyro, measurement_angle)


%-------------------------------
%-------------------------------
%---- Predict Stage ------------
%-------------------------------
%-------------------------------
% pix_value = 5;
Ts = 1/400;
%Process Noise
p_var =0.01;
Q = [p_var^2     0         
      0         p_var^2];

%A matrix
A =  [1   -Ts 
      0   1];

%odutput these values with a unit delay (for algebraic loop), apply initial conditions
state_prediction = A*prev_state + [Ts 0; 0 0]*[ctrl_input_gyro; 0 ];
covariance_prediction = A*covariance_correction_prev*A' + Q;

%-------------------------------
%-------------------------------
%---- Estimate Stage -----------
%-------------------------------
%-------------------------------

    %H matrix
    H = [1 0];

    %Measurement noise from accelerometer angle measurement
    m_var = 0.5;
%     m_var_r = 1;

    R = [m_var^2 ];

    %Measurement Z
    Z = [measurement_angle];

    %Compute Kalman Gain
    Kalman_Gain = covariance_prediction*H'*inv(H*covariance_prediction*H'+R); %2x2 matrix

    %compute state space correction based on measurement
    state_correction = state_prediction + Kalman_Gain*(Z - H*state_prediction); %4x1 vector of states

    %compute covariance correction
    covariance_correction = (eye(2) - Kalman_Gain*H)*covariance_prediction; %2x2 covariance matrix

%     corrected_angle_measure = state_correction(1) - Ts*state_correction(2);
end

== matlab function Record_accelerometer/Navigation Subsystem/KF_PITCH/Kalman Tracker ==
  data: prev_state input; covariance_correction_prev input; state_correction output; covariance_correction output; ctrl_input_gyro input; measurement_angle input
function [state_correction, covariance_correction] = fcn(prev_state, covariance_correction_prev, ctrl_input_gyro, measurement_angle)


%-------------------------------
%-------------------------------
%---- Predict Stage ------------
%-------------------------------
%-------------------------------
% pix_value = 5;
Ts = 1/400;
%Process Noise
p_var =0.01;
Q = [p_var^2     0         
      0         p_var^2];

%A matrix
A =  [1   -Ts 
      0   1];

%odutput these values with a unit delay (for algebraic loop), apply initial conditions
state_prediction = A*prev_state + [Ts 0; 0 0]*[ctrl_input_gyro; 0 ];
covariance_prediction = A*covariance_correction_prev*A' + Q;

%-------------------------------
%-------------------------------
%---- Estimate Stage -----------
%-------------------------------
%-------------------------------

    %H matrix
    H = [1 0];

    %Measurement noise from accelerometer angle measurement
    m_var = 1;
%     m_var_r = 1;

    R = [m_var^2 ];

    %Measurement Z
    Z = [measurement_angle];

    %Compute Kalman Gain
    Kalman_Gain = covariance_prediction*H'*inv(H*covariance_prediction*H'+R); %2x2 matrix

    %compute state space correction based on measurement
    state_correction = state_prediction + Kalman_Gain*(Z - H*state_prediction); %4x1 vector of states

    %compute covariance correction
    covariance_correction = (eye(2) - Kalman_Gain*H)*covariance_prediction; %2x2 covariance matrix

%     corrected_angle_measure = state_correction(1) - Ts*state_correction(2);
end
